simulink model "CP_ContrSys_Lin_b_n9329013"  (R2017b)
settings: Solver=ode4  StartTime=0.0  StopTime=10.0  FixedStep=0.02  RelTol=1e-3
values from neighbouring files (symbols this model uses):
  A = [0,0,1,0;0,0,0,1;0,((-m*g)/(Mc)),0,0;0,((g*(Mc+m))/(l*Mc)),0,0]    [CP_ContrSys_Lin_a_Mainfile_n9329013.m]    (also in CP_ContrSys_Lin_b_Mainfile_n9329013.m = [0,0,1,0;0,0,0,1;0,((-m*g)/(Mc)),0,0;0,-((g*(Mc+m))/(l*Mc)),; EGH445_Computer_Lab_1.m = [0,2,-8;3,5,4;-1.5,-1,1]; MainFile_Linearised_a_9329013.m; MainFile_Linearised_b_9329013.m = [0,0,1,0;0,0,0,1;0,((-m*g)/(Mc)),0,0;0,-((g*(Mc+m))/(l*Mc)),)
  B = [0,0,(1/Mc),-((1)/(l*Mc))]'    [CP_ContrSys_Lin_a_Mainfile_n9329013.m]    (also in CP_ContrSys_Lin_b_Mainfile_n9329013.m = [0,0,(1/Mc),((1)/(l*Mc))]'; EGH445_Computer_Lab_1.m = [4,4,0;1,4,0;-1,-2,2]; MainFile_Linearised_a_9329013.m; MainFile_Linearised_b_9329013.m = [0,0,(1/Mc),((1)/(l*Mc))]')
  C = eye(4)    [CP_ContrSys_Lin_a_Mainfile_n9329013.m]    (also in CP_ContrSys_Lin_b_Mainfile_n9329013.m; MainFile_Linearised_a_9329013.m; MainFile_Linearised_b_9329013.m)
  CObs = [1,0,0,0;0,1,0,0]    [CP_ContrSys_Lin_a_Mainfile_n9329013.m]    (also in CP_ContrSys_Lin_b_Mainfile_n9329013.m)
  D = zeros(4,1)    [CP_ContrSys_Lin_a_Mainfile_n9329013.m]    (also in CP_ContrSys_Lin_b_Mainfile_n9329013.m; MainFile_Linearised_a_9329013.m; MainFile_Linearised_b_9329013.m)
  Lb = place(A',CObs',observer_error_dynamics)'    [CP_ContrSys_Lin_b_Mainfile_n9329013.m]
undefined symbols (not defined in the file or in its folder): Kb
settings Model: Creator=Koh Kim Hai  LastModifiedBy=Koh Kim Hai
settings DataIOCC: TimeSaveName=toutb_tilde
settings OptimizationCC: BlockReduction=off  DefaultParameterBehavior=Inlined  BufferReuse=off

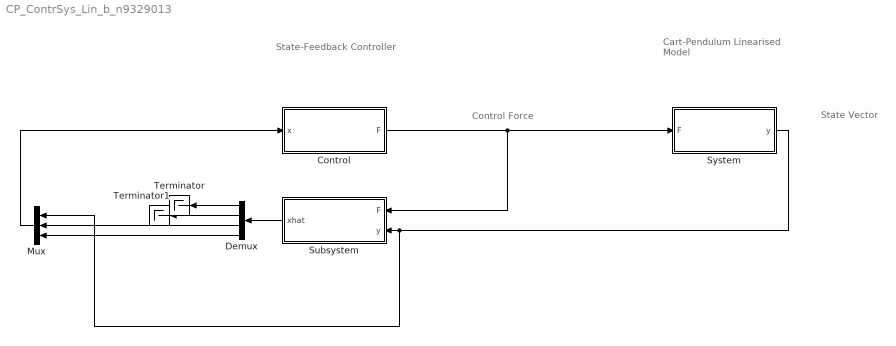
== system CP_ContrSys_Lin_b_n9329013 ==
  note: State Vector
  note: Control Force
  note: State-Feedback Controller
  note: Cart-Pendulum Linearised Model
  Control : Subsystem
  Demux : Demux
  Mux : Mux  Inputs=3
  Subsystem : Subsystem
  System : Subsystem
  Terminator : Terminator
  Terminator1 : Terminator
  wires:
  System/1(y) -> Mux/1, Subsystem/2(y)
  Control/1(F) -> Subsystem/1(F), System/1(F)
  Subsystem/1(xhat) -> Demux/1
  Demux/1 -> Terminator/1
  Demux/2 -> Terminator1/1
  Demux/3 -> Mux/2
  Demux/4 -> Mux/3
  Mux/1 -> Control/1(x)

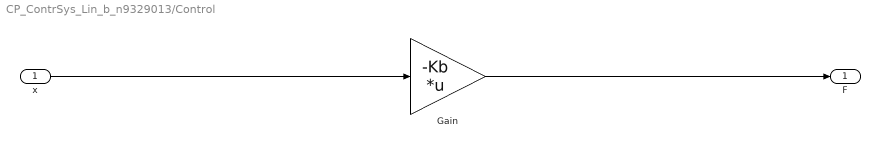
== system CP_ContrSys_Lin_b_n9329013/Control ==
  x : Inport
  Gain : Gain  Gain=-Kb  Multiplication=Matrix(K*u)
  F : Outport
  wires:
  x/1 -> Gain/1
  Gain/1 -> F/1

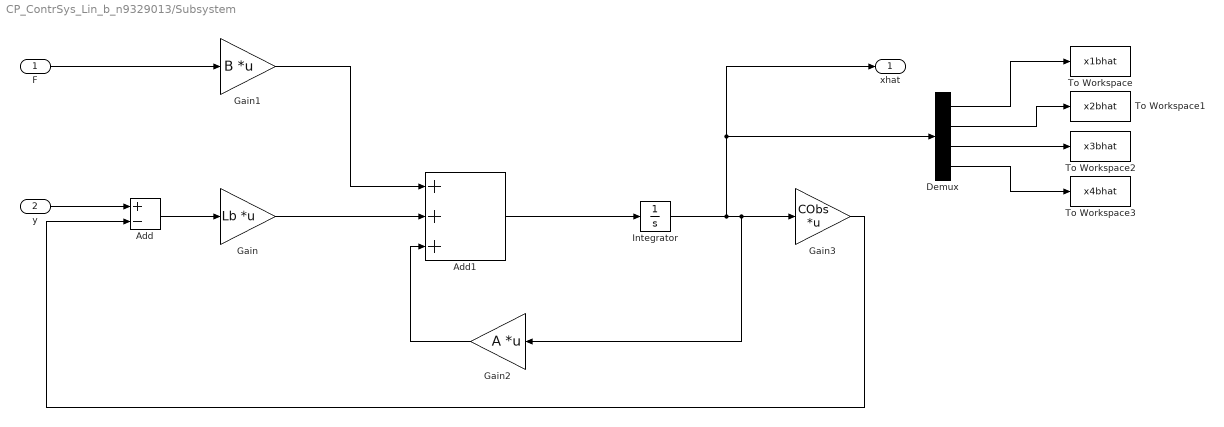
== system CP_ContrSys_Lin_b_n9329013/Subsystem ==
  F : Inport
  y : Inport  Port=2
  Add : Sum  Inputs=+-
  Add1 : Sum  Inputs=+++
  Demux : Demux
  Gain : Gain  Gain=Lb  Multiplication=Matrix(K*u)
  Gain1 : Gain  Gain=B  Multiplication=Matrix(K*u)
  Gain2 : Gain  Gain=A  Multiplication=Matrix(K*u)
  Gain3 : Gain  Gain=CObs  Multiplication=Matrix(K*u)
  Integrator : Integrator
  To Workspace : ToWorkspace  VariableName=x1bhat  SampleTime=-1
  To Workspace1 : ToWorkspace  VariableName=x2bhat  SampleTime=-1
  To Workspace2 : ToWorkspace  VariableName=x3bhat  SampleTime=-1
  To Workspace3 : ToWorkspace  VariableName=x4bhat  SampleTime=-1
  xhat : Outport
  wires:
  y/1 -> Add/1
  Add/1 -> Gain/1
  Gain1/1 -> Add1/1
  Gain/1 -> Add1/2
  Gain2/1 -> Add1/3
  Add1/1 -> Integrator/1
  Integrator/1 -> Demux/1, xhat/1, Gain2/1, Gain3/1
  Gain3/1 -> Add/2
  Demux/1 -> To Workspace/1
  Demux/2 -> To Workspace1/1
  Demux/3 -> To Workspace2/1
  Demux/4 -> To Workspace3/1
  F/1 -> Gain1/1

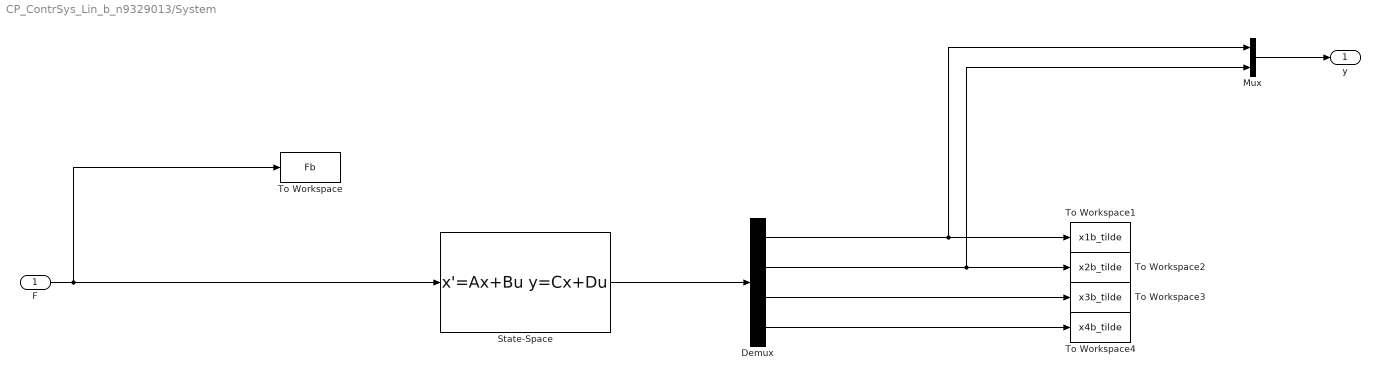
== system CP_ContrSys_Lin_b_n9329013/System ==
  F : Inport
  Demux : Demux
  Mux : Mux  Inputs=2
  State-Space : StateSpace  A=A  B=B  C=C  D=D  InitialCondition=[0.2,20*pi/180,0,0]'
  To Workspace : ToWorkspace  VariableName=Fb  SampleTime=-1
  To Workspace1 : ToWorkspace  VariableName=x1b_tilde  SampleTime=-1
  To Workspace2 : ToWorkspace  VariableName=x2b_tilde  SampleTime=-1
  To Workspace3 : ToWorkspace  VariableName=x3b_tilde  SampleTime=-1
  To Workspace4 : ToWorkspace  VariableName=x4b_tilde  SampleTime=-1
  y : Outport
  wires:
  Demux/1 -> Mux/1, To Workspace1/1
  F/1 -> State-Space/1, To Workspace/1
  Demux/2 -> To Workspace2/1, Mux/2
  Demux/3 -> To Workspace3/1
  Demux/4 -> To Workspace4/1
  State-Space/1 -> Demux/1
  Mux/1 -> y/1
